simulink model "MSDRL"  (R2024b)
settings: Solver=VariableStepAuto  StartTime=0.0  StopTime=10.0  RelTol=1e-3
values from neighbouring files (symbols this model uses):
  v0 = 0    [msdResetFcn.m]
  x0 = 0    [msdResetFcn.m]
libraries: simulink x1, rllib x1
settings Model: Creator=Robin  LastModifiedBy=Robin

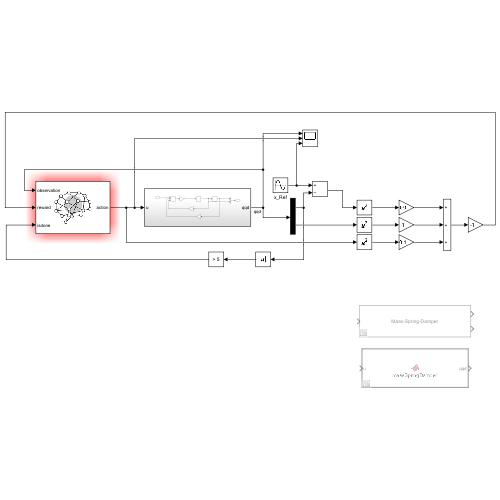
[thumbnail: Simulink's stored preview of the top-level diagram]
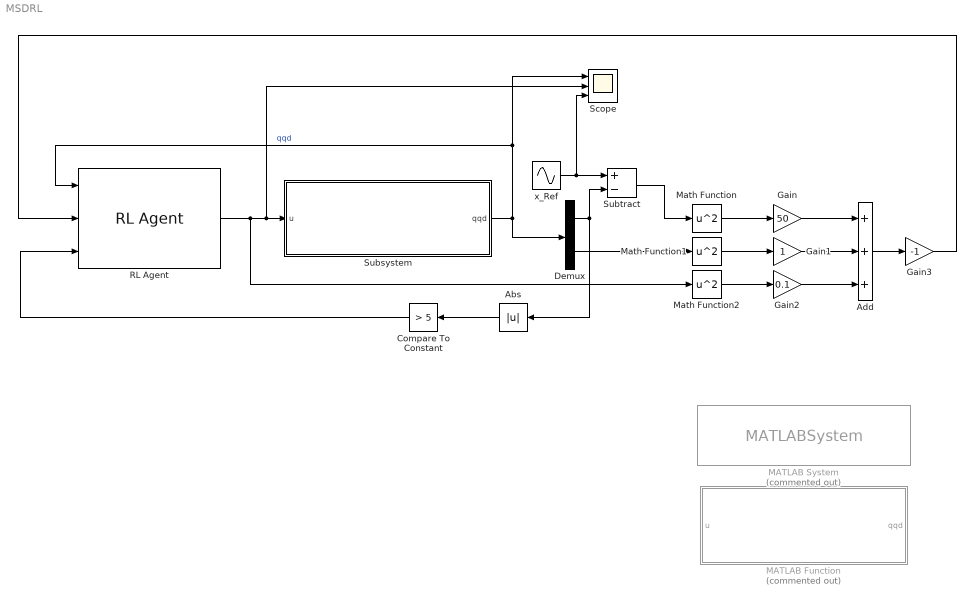
== system MSDRL ==
  Abs : Abs  SaturateOnIntegerOverflow=off
  Add : Sum  Inputs=+++
  Compare To Constant : simulink/Logic and Bit Operations/Compare To Constant  relop=>  const=5  OutDataTypeStr=boolean
  Demux : Demux  Outputs=2
  Gain : Gain  Gain=50
  Gain1 : Gain
  Gain2 : Gain  Gain=0.1
  Gain3 : Gain  Gain=-1
  MATLAB Function : MATLAB Function  Commented=on  TreatAsAtomicUnit=on  SystemSampleTime=0.01
  MATLAB System : MATLABSystem  Commented=on  System=MSDSystem  m=1  c=0.5  k=10  SimulateUsing=Code generation
      mask Type: MSDSystem
      mask Display: disp('Mass-Spring-Damper');
  Math Function : Math  Operator=square
  Math Function1 : Math  Operator=square
  Math Function2 : Math  Operator=square
  RL Agent : rllib/RL Agent  Agent=agent  ExternalActionAsInput=off  ProvideLastAction=off  ProvideCumRwd=off  TreatAsDirectFeedthrough=on  UseStrictObservationDataTypes=off
  Scope : Scope  NumInputPorts=3
  Subsystem : Subsystem
  Subtract : Sum  Inputs=+-
  x_Ref : Sin  SampleTime=0
  wires:
  RL Agent/1 -> Math Function2/1, Scope/2, Subsystem/1(u)
  Subsystem/1(qqd) -> Demux/1, Scope/1, RL Agent/1  "qqd"
  Demux/1 -> Subtract/2, Abs/1
  Demux/2 -> Math Function1/1
  Math Function/1 -> Gain/1
  Math Function1/1 -> Gain1/1
  Math Function2/1 -> Gain2/1
  Gain/1 -> Add/1
  Gain1/1 -> Add/2
  Gain2/1 -> Add/3
  Add/1 -> Gain3/1
  Gain3/1 -> RL Agent/2
  Abs/1 -> Compare To Constant/1
  Compare To Constant/1 -> RL Agent/3
  x_Ref/1 -> Scope/3, Subtract/1
  Subtract/1 -> Math Function/1

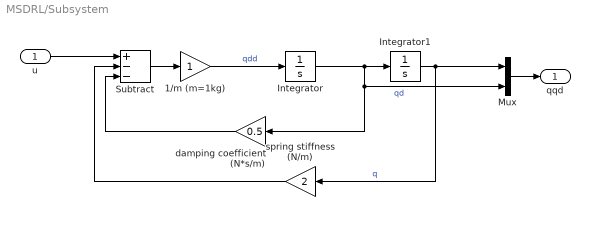
== system MSDRL/Subsystem ==
  u : Inport
  1/m (m=1kg) : Gain
  Integrator : Integrator  InitialCondition=v0
  Integrator1 : Integrator  InitialCondition=x0
  Mux : Mux  Inputs=2
  Subtract : Sum  Inputs=+--
  damping coefficient (N*s/m) : Gain  Gain=0.5
  spring stiffness (N/m) : Gain  Gain=2
  qqd : Outport
  wires:
  u/1 -> Subtract/1
  1/m (m=1kg)/1 -> Integrator/1  "qdd"
  Subtract/1 -> 1/m (m=1kg)/1
  Integrator/1 -> damping coefficient (N*s/m)/1, Mux/2, Integrator1/1  "qd"
  Integrator1/1 -> Mux/1, spring stiffness (N/m)/1  "q"
  damping coefficient (N*s/m)/1 -> Subtract/3
  spring stiffness (N/m)/1 -> Subtract/2
  Mux/1 -> qqd/1

== matlab function MSDRL/MATLAB Function ==
  settings: updateMethod=DISCRETE
  data: u input; qqd output
function qqd = massSpringDamper(u)
% Continuous-time mass-spring-damper system
% u: input force (N)
% pos: output position (m)
% vel: output velocity (m/s)

%% system paramters
m = 1.0;    % Mass (kg
c = 0.5;    % Damping coefficient (Ns/m)
k = 2.0;    % Spring stiffness (N/m)
Ts = 0.01;  % Sample time(s)

%% Persistent state variables
persistent q_prev
if isempty(q_prev)
    q_prev = [0, 0]; % Initial condition [position, velocity]
end

%% Compute acceleration
qdd = (u - c * q_prev(2) - k * q_prev(1)) / m;

%% update states using Euler integration
qd = q_prev(2) + Ts * qdd;
q = q_prev(1) + Ts * qd;

%% Update persistent variables
q_prev = [q, qd];

%% Output;
qqd = q_prev;
